simulink subsystem "ReferenceOutputSafetyLimitation"  (R2024b)
settings: Solver=VariableStepAuto  StartTime=0.0  StopTime=10.0  RelTol=1e-3
undefined symbols (not defined in the file): voltSEPICMax
libraries: simulink x1
settings Model: DefaultTestHarness=Supervisory_Logic_Harness1  Creator=vlenzi  LastModifiedBy=vlenzi
settings RTWCC: GPUComputeCapability=3.5

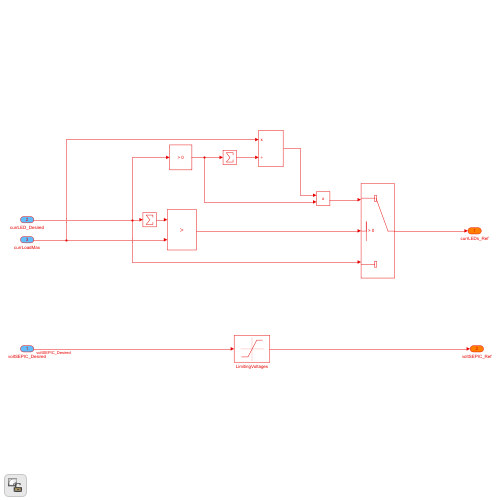
[thumbnail: Simulink's stored preview of the top-level diagram]
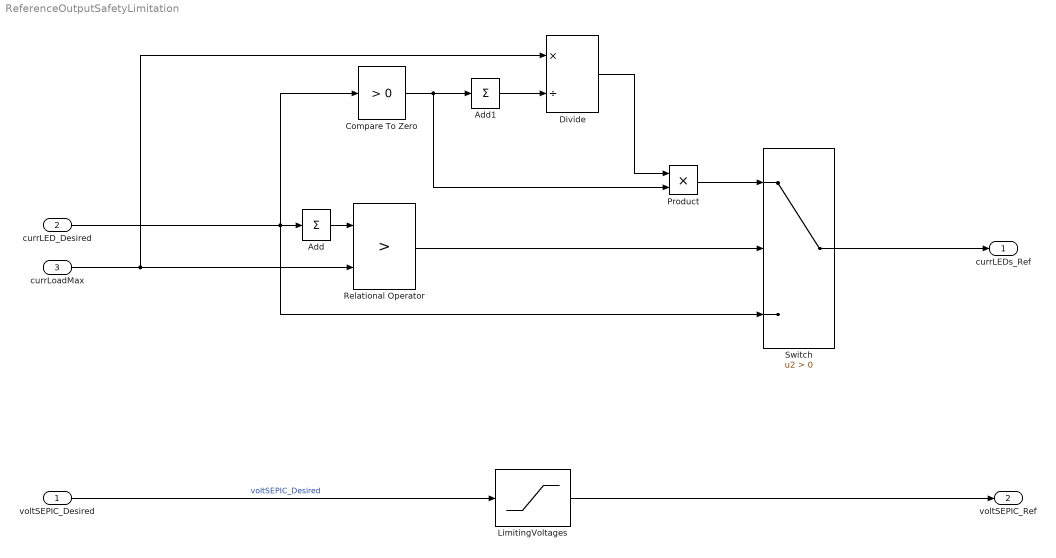
== system ReferenceOutputSafetyLimitation ==
  voltSEPIC_Desired : Inport  OutDataTypeStr=single  PortDimensions=1
  currLED_Desired : Inport  Port=2
  currLoadMax : Inport  Port=3
  Add : Sum  Inputs=+
  Add1 : Sum  Inputs=+
  Compare To Zero : simulink/Logic and Bit Operations/Compare To Zero  relop=>  OutDataTypeStr=boolean
  Divide : Product  Inputs=*/
  LimitingVoltages : Saturate  UpperLimit=voltSEPICMax  LowerLimit=0
  Product : Product
  Relational Operator : RelationalOperator  Operator=>  OutDataTypeStr=boolean  RndMeth=Simplest  InputSameDT=off
  Switch : Switch  Criteria=u2 > Threshold  SaturateOnIntegerOverflow=off  InputSameDT=off
  currLEDs_Ref : Outport
  voltSEPIC_Ref : Outport  Port=2  OutDataTypeStr=single  PortDimensions=1
  wires:
  Add/1 -> Relational Operator/1
  currLED_Desired/1 -> Switch/3, Compare To Zero/1, Add/1
  currLoadMax/1 -> Divide/1, Relational Operator/2
  Relational Operator/1 -> Switch/2
  Switch/1 -> currLEDs_Ref/1
  Compare To Zero/1 -> Add1/1, Product/2
  Add1/1 -> Divide/2
  Product/1 -> Switch/1
  Divide/1 -> Product/1
  voltSEPIC_Desired/1 -> LimitingVoltages/1  "voltSEPIC_Desired"
  LimitingVoltages/1 -> voltSEPIC_Ref/1
